simulink model "LWR4_ElasticJoints"  (R2014a)
settings: Solver=ode23tb  StartTime=0.0  StopTime=10  RelTol=1e-6  AbsTol=1e-6
values from neighbouring files (symbols this model uses):
  ACTIVATE_COULOMB_FRICTION = 0    [loadparam.m]
  B = Km*diag([im1 im2 im3 im4 im5 im6 im7])*Km    [loadparam.m]
  eta = 0.95    [loadparam.m]
  Ki = 15*eye(7)    [loadparam.m]
  Kj = diag([1e4 1e4 1e4 1e4 1e4 7.5e3 7.5e3])    [loadparam.m]
  Km = diag([km1 km2 km3 km4 km5 km6 km7])    [loadparam.m]
  NominalDynamicParameters = [il1x il1y il1z il2x il2y il2z il3x il3y il3z il4x il4y il4z il5x il5y il5z il6x il6y il6z il7x il7y il7z                             g pl1y pl2z pl3y pl4z pl5y pl7z pm1z pm3z pm5z im1 im2 im3 im4 im5 im6 im7                             fv1 fv2 fv3 fv4 fv5 fv6 fv7 fc1 fc2 fc3 fc4 fc5 fc6 fc7]    [DefineNominalParameters.m]    (also in loadparam.m = DefineNominalParameters(d0,d3,d5,d7,r1,r2,r3,r4,r5,r6,r7,h7,)
  omegaT = 1e-3    (= 0.001)    [loadparam.m]
  q0 = [0 pi/2-0.3 0 0.3 0 0 0]'    [loadparam.m]
  Ts = 2e-3    (= 0.002)    [loadparam.m]
  UncertainDynamicParameters = [il1x il1y il1z il2x il2y il2z il3x il3y il3z il4x il4y il4z il5x il5y il5z il6x il6y il6z il7x il7y il7z                               g pl1y pl2z pl3y pl4z pl5y pl7z pm1z pm3z pm5z im1 im2 im3 im4 im5 im6 im7                               fv1 fv2 fv3 fv4 fv5 fv6 fv7 fc1 fc2 fc3 fc4 fc5 fc6 fc7]    [DefineUncertainParameters.m]    (also in loadparam.m = NominalDynamicParameters)
settings Model: Creator=Ciro  LastModifiedBy=Ciro
settings DataIOCC: SignalLoggingSaveFormat=ModelDataLogs
settings OptimizationCC: ExpressionDepthLimit=2147483647
settings DebuggingCC: UnderspecifiedInitializationDetection=Classic  FcnCallInpInsideContextMsg=EnableAllAsWarning  StateNameClashWarn=warning

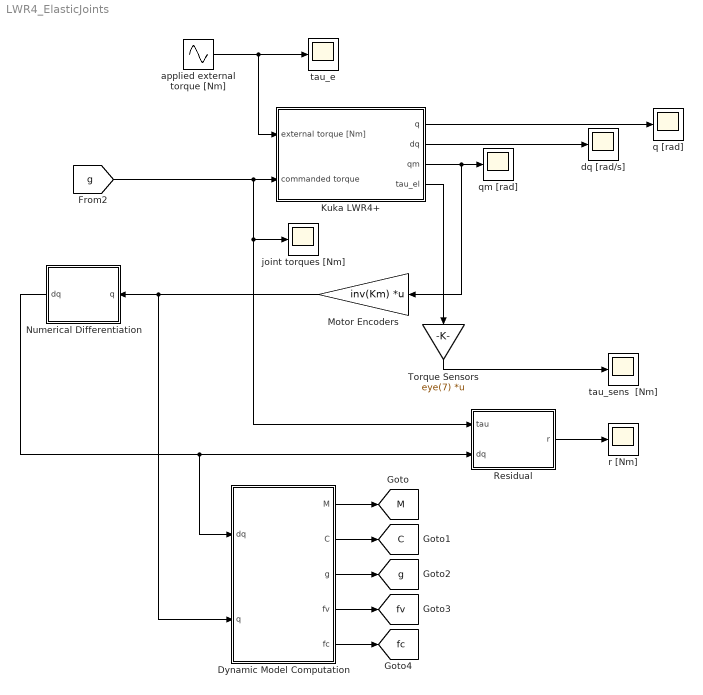
== system LWR4_ElasticJoints ==
  Dynamic Model Computation : MATLAB Function  TreatAsAtomicUnit=on
  Kuka LWR4+ : Subsystem
      mask Display: image(imread('lwr4.jpg'))
  Motor Encoders : Gain  Gain=inv(Km)  Multiplication=Matrix(K*u)  SampleTime=Ts
  Numerical Differentiation : Subsystem
  Residual : Subsystem
  Torque Sensors : Gain  Gain=eye(7)  Multiplication=Matrix(K*u)  SampleTime=Ts
  applied external torque [Nm] : Sin  Amplitude=[10 0 0 7 0 4 0]*0.5  Frequency=2*pi*0.25  SampleTime=0
  dq [rad/s] : Scope
      settings: YMin=-0.5  YMax=0.6  SaveName=dq  SampleInput=on  SampleTime=Ts
  joint torques [Nm] : Scope
      settings: YMin=-30  SaveName=u  SampleInput=on  SampleTime=Ts
  q [rad] : Scope
      settings: YMin=-0.25  YMax=3.25  SaveName=q  SampleInput=on  SampleTime=Ts
  qm [rad] : Scope
      settings: YMin=-250  YMax=125  SaveName=qm  SampleInput=on  SampleTime=Ts
  r [Nm] : Scope
      settings: TimeRange=10  YMin=-10  YMax=10  SaveName=r  SampleInput=on  SampleTime=Ts
  tau_e : Scope
      settings: YMin=0  SaveName=tau_e  SampleInput=on  SampleTime=Ts
  tau_sens  [Nm] : Scope
      settings: YMin=-90  YMax=10  SaveName=r1  SampleInput=on  SampleTime=Ts
  tag scope: C=global, M=global, fc=global, fv=global, g=global
  wires:
  Kuka LWR4+/1(q) -> q [rad]/1
  Kuka LWR4+/2(dq) -> dq [rad/s]/1
  Kuka LWR4+/3(qm) -> Motor Encoders/1, qm [rad]/1
  applied external torque [Nm]/1 -> tau_e/1, Kuka LWR4+/1(external torque [Nm])
  [g] -> Kuka LWR4+/2(commanded torque), joint torques [Nm]/1, Residual/1(tau)
  Numerical Differentiation/1(dq) -> Dynamic Model Computation/1(dq), Residual/2(dq)
  Residual/1(r) -> r [Nm]/1
  Kuka LWR4+/4(tau_el) -> Torque Sensors/1
  Dynamic Model Computation/1(M) -> [M]
  Dynamic Model Computation/2(C) -> [C]
  Dynamic Model Computation/3(g) -> [g]
  Dynamic Model Computation/4(fv) -> [fv]
  Dynamic Model Computation/5(fc) -> [fc]
  Torque Sensors/1 -> tau_sens  [Nm]/1
  Motor Encoders/1 -> Dynamic Model Computation/2(q), Numerical Differentiation/1(q)

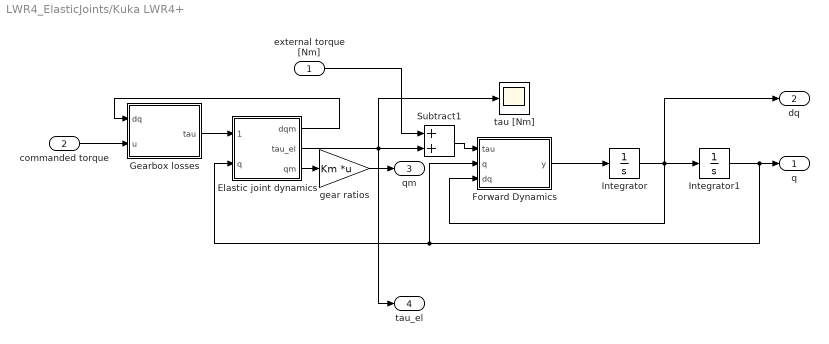
== system LWR4_ElasticJoints/Kuka LWR4+ ==
  external torque [Nm] : Inport
  commanded torque : Inport  Port=2
  Elastic joint dynamics : Subsystem
  Forward Dynamics : MATLAB Function  TreatAsAtomicUnit=on
  Gearbox losses : MATLAB Function  TreatAsAtomicUnit=on
  Integrator : Integrator  InitialCondition=zeros(7,1)
  Integrator1 : Integrator  InitialCondition=q0
  Subtract1 : Sum
  gear ratios : Gain  Gain=Km  Multiplication=Matrix(K*u)
  tau [Nm] : Scope
      settings: YMin=-250  YMax=125  SaveName=tau  SampleTime=Ts
  q : Outport
  dq : Outport  Port=2
  qm : Outport  Port=3
  tau_el : Outport  Port=4
  wires:
  Integrator/1 -> Integrator1/1, Forward Dynamics/3(dq), dq/1
  Forward Dynamics/1(y) -> Integrator/1
  Integrator1/1 -> q/1, Forward Dynamics/2(q), Elastic joint dynamics/2(q)
  Gearbox losses/1(tau) -> Elastic joint dynamics/1(tau_m)
  Elastic joint dynamics/1(dqm) -> Gearbox losses/1(dq)
  Elastic joint dynamics/2(tau_el) -> tau_el/1, tau [Nm]/1, Subtract1/2
  commanded torque/1 -> Gearbox losses/2(u)
  Elastic joint dynamics/3(qm) -> gear ratios/1
  gear ratios/1 -> qm/1
  Subtract1/1 -> Forward Dynamics/1(tau)
  external torque [Nm]/1 -> Subtract1/1

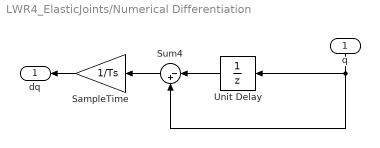
== system LWR4_ElasticJoints/Numerical Differentiation ==
  q : Inport
  SampleTime : Gain  Gain=1/Ts  SampleTime=Ts
  Sum4 : Sum  Inputs=|-+
  Unit Delay : UnitDelay  InitialCondition=q0  SampleTime=Ts
  dq : Outport
  wires:
  Unit Delay/1 -> Sum4/1
  Sum4/1 -> SampleTime/1
  q/1 -> Unit Delay/1, Sum4/2
  SampleTime/1 -> dq/1

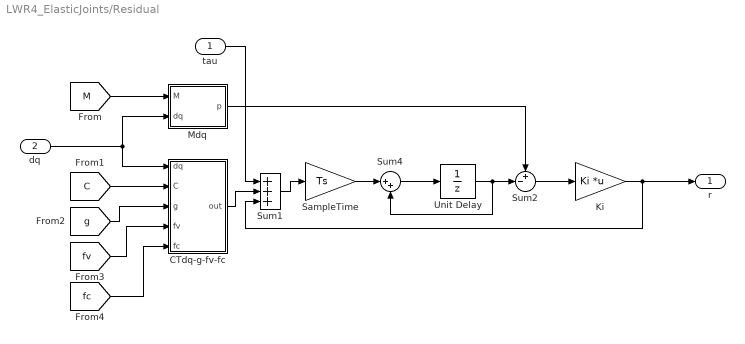
== system LWR4_ElasticJoints/Residual ==
  tau : Inport
  dq : Inport  Port=2
  CTdq-g-fv-fc : MATLAB Function  TreatAsAtomicUnit=on
  Ki : Gain  Gain=Ki  Multiplication=Matrix(K*u)  SampleTime=Ts
  Mdq : MATLAB Function  TreatAsAtomicUnit=on
  SampleTime : Gain  Gain=Ts  SampleTime=Ts
  Sum1 : Sum  Inputs=+++
  Sum2 : Sum  Inputs=+-|
  Sum4 : Sum  Inputs=|++
  Unit Delay : UnitDelay  InitialCondition=zeros(7,1)  SampleTime=Ts
  r : Outport
  wires:
  tau/1 -> Sum1/1
  Sum2/1 -> Ki/1
  CTdq-g-fv-fc/1(out) -> Sum1/2
  Mdq/1(p) -> Sum2/1
  Sum1/1 -> SampleTime/1
  Sum4/1 -> Unit Delay/1
  SampleTime/1 -> Sum4/1
  Ki/1 -> r/1, Sum1/3
  Unit Delay/1 -> Sum2/2, Sum4/2
  dq/1 -> Mdq/2(dq), CTdq-g-fv-fc/1(dq)
  [M] -> Mdq/1(M)
  [C] -> CTdq-g-fv-fc/2(C)
  [g] -> CTdq-g-fv-fc/3(g)
  [fv] -> CTdq-g-fv-fc/4(fv)
  [fc] -> CTdq-g-fv-fc/5(fc)

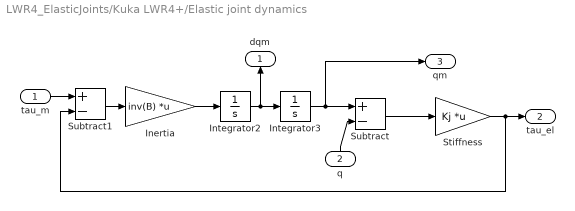
== system LWR4_ElasticJoints/Kuka LWR4+/Elastic joint dynamics ==
  tau_m : Inport
  q : Inport  Port=2
  Inertia : Gain  Gain=inv(B)  Multiplication=Matrix(K*u)
  Integrator2 : Integrator  InitialCondition=zeros(7,1)
  Integrator3 : Integrator  InitialCondition=q0
  Stiffness : Gain  Gain=Kj  Multiplication=Matrix(K*u)
  Subtract : Sum  Inputs=+-
  Subtract1 : Sum  Inputs=+-
  dqm : Outport
  tau_el : Outport  Port=2
  qm : Outport  Port=3
  wires:
  Integrator2/1 -> Integrator3/1, dqm/1
  Stiffness/1 -> Subtract1/2, tau_el/1
  Subtract/1 -> Stiffness/1
  Integrator3/1 -> Subtract/1, qm/1
  Inertia/1 -> Integrator2/1
  Subtract1/1 -> Inertia/1
  q/1 -> Subtract/2
  tau_m/1 -> Subtract1/1

== matlab function LWR4_ElasticJoints/Kuka LWR4+/Gearbox losses ==
  data: dq input; tau output; u input; eta parameter; omegaT parameter
function tau = losses(dq,u,eta,omegaT)
%#codegen

% Computes the torque losses in the gearboxes
%
% function tau = torque_losses(u,dq)
%
% input:
%       u     dim 7x1     motor torques
%       dq    dim 7x1     joint velocities
%
% output:
%       tau   dim 7x1     actual joint torques
%
% parameters:
%       eta    dim 1x1     efficiency of the gearbox (<1)
%       omegaT dim 1x1     threshold motor speed for regularization purposes
%
% G. Antonelli, Sistemi Robotici, fall 2012

tau = u -(1-eta)*abs(u).*tanh(4/omegaT*dq);

== matlab function LWR4_ElasticJoints/Kuka LWR4+/Forward Dynamics ==
  data: tau input; q input; y output; dq input; UncertainDynamicParameters parameter; ACTIVATE_COULOMB_FRICTION parameter
function y = ddq(tau,q,dq,UncertainDynamicParameters,ACTIVATE_COULOMB_FRICTION)
%#codegen

% Computes the direct dynamics for the Kuka LWR
%
% function y = ddq(tau,dq,q,UncertainDynamicParameters,ACTIVATE_COULOMB_FRICTION)
%
% input:
%       tau     dim 7x1     joint torques
%       dq      dim 7x1     joint velocities
%       q       dim 7x1     joint positions
%       UncertainDynamicParameters dim 52x1    dynamic parameters subject to uncertainties
%       ACTIVATE_COULOMB_FRICTION: flag to activate (1) or deactivate (0) Coulomb dry friction
%
% output:
%       y     dim 7x1     joint accelerations
%
% G. Antonelli, Sistemi Robotici, fall 2012
% Revised: C. Natale, February 2015

g = gravity(q,UncertainDynamicParameters);

Cdq = CoriolisMatrix(q,dq,UncertainDynamicParameters)*dq;

fv1 = UncertainDynamicParameters(39);
fv2 = UncertainDynamicParameters(40);
fv3 = UncertainDynamicParameters(41);
fv4 = UncertainDynamicParameters(42);
fv5 = UncertainDynamicParameters(43);
fv6 = UncertainDynamicParameters(44);
fv7 = UncertainDynamicParameters(45);
fc1 = UncertainDynamicParameters(46);
fc2 = UncertainDynamicParameters(47);
fc3 = UncertainDynamicParameters(48);
fc4 = UncertainDynamicParameters(49);
fc5 = UncertainDynamicParameters(50);
fc6 = UncertainDynamicParameters(51);
fc7 = UncertainDynamicParameters(52);
Fv=diag([fv1 fv2 fv3 fv4 fv5 fv6 fv7]);
Fc=diag([fc1 fc2 fc3 fc4 fc5 fc6 fc7]);

f = Fv*dq+ACTIVATE_COULOMB_FRICTION*Fc*sign(dq);

M = InertiaMatrix(q,UncertainDynamicParameters);

y = M\(tau - g - Cdq - f);

== matlab function LWR4_ElasticJoints/Residual/Mdq ==
  data: M input; dq input; p output
function p = Mdq(M,dq)
%#codegen

p = M*dq;

== matlab function LWR4_ElasticJoints/Residual/CTdq-g-fv-fc ==
  data: dq input; C input; g input; out output; fv input; fc input
function out = nonlin(dq,C,g,fv,fc)
%#codegen

out = C'*dq-g-fv-fc;

== matlab function LWR4_ElasticJoints/Dynamic Model Computation ==
  data: dq input; q input; NominalDynamicParameters parameter; M output; ACTIVATE_COULOMB_FRICTION parameter; C output; g output; fv output; fc output
function [M,C,g,fv,fc] = DynamicModel(dq,q,NominalDynamicParameters,ACTIVATE_COULOMB_FRICTION)
%#codegen

fv1 = NominalDynamicParameters(39);
fv2 = NominalDynamicParameters(40);
fv3 = NominalDynamicParameters(41);
fv4 = NominalDynamicParameters(42);
fv5 = NominalDynamicParameters(43);
fv6 = NominalDynamicParameters(44);
fv7 = NominalDynamicParameters(45);
fc1 = NominalDynamicParameters(46);
fc2 = NominalDynamicParameters(47);
fc3 = NominalDynamicParameters(48);
fc4 = NominalDynamicParameters(49);
fc5 = NominalDynamicParameters(50);
fc6 = NominalDynamicParameters(51);
fc7 = NominalDynamicParameters(52);
Fv=diag([fv1 fv2 fv3 fv4 fv5 fv6 fv7]);
Fc=diag([fc1 fc2 fc3 fc4 fc5 fc6 fc7]);


fv = Fv*dq;

fc = ACTIVATE_COULOMB_FRICTION*Fc*sign(dq);

C = CoriolisMatrix(q,dq,NominalDynamicParameters);

g = gravity(q,NominalDynamicParameters);

M = InertiaMatrix(q,NominalDynamicParameters);
